simulink model "modello"  (R2022b)
settings: Solver=VariableStepAuto  StartTime=0.0  StopTime=tfinal  RelTol=1e-3
values from neighbouring files (symbols this model uses):
  A1 = [0.361538461538 0.0769230769231 0.153846153846 0.307692307692 0.272727272727 0.0818181818182 0.181818181818 0.363636363636 0.25 0.0833333333333 0.233333333333 0.333333333333 ... (16 elements, 4x4)]    [data_sim.mat]    (also in model_matrices.m = A)
  A2 = [0.4 0 0 0 0 0.5 0 0 0.4 0 0 0 ... (49 elements, 7x7)]    [data_sim.mat]    (also in model_matrices.m = A)
  A3 = [0.3 0.3 0.1 0.1 0.1 0.222222222222 0.566666666667 0 0 0.111111111111 0.5 0 ... (25 elements, 5x5)]    [data_sim.mat]    (also in model_matrices.m = A)
  A4 = [0.531578947368 0.105263157895 0.105263157895 0.105263157895 0.0526315789474 0.6 0.3 0 0 0 0.6 0 ... (25 elements, 5x5)]    [data_sim.mat]    (also in model_matrices.m = A)
  A5 = [0.566666666667 0.111111111111 0.111111111111 0.111111111111 0.6 0.3 0 0 0.5 0 0.233333333333 0.166666666667 ... (16 elements, 4x4)]    [data_sim.mat]    (also in model_matrices.m = A)
  a_0i = 0.1    [data_sim.mat]    (also in model_matrices.m)
  B1 = [1 0 0 0 0 1 0 0 0 0 1 0 ... (16 elements, 4x4)]    [data_sim.mat]    (also in model_matrices.m = eye(4))
  B2 = [1 0 0 0 0 0 0 0 1 0 0 0 ... (49 elements, 7x7)]    [data_sim.mat]    (also in model_matrices.m = eye(rn2))
  B3 = [1 0 0 0 0 0 1 0 0 0 0 0 ... (25 elements, 5x5)]    [data_sim.mat]    (also in model_matrices.m = eye(rn3))
  B4 = [1 0 0 0 0 0 1 0 0 0 0 0 ... (25 elements, 5x5)]    [data_sim.mat]    (also in model_matrices.m = eye(rn4))
  B5 = [1 0 0 0 0 1 0 0 0 0 1 0 ... (16 elements, 4x4)]    [data_sim.mat]    (also in model_matrices.m = eye(rn5))
  C1 = [1 0 0 0 0 1 0 0 0 0 1 0 ... (16 elements, 4x4)]    [data_sim.mat]    (also in model_matrices.m = eye(4))
  C2 = [1 0 0 0 0 0 0 0 1 0 0 0 ... (49 elements, 7x7)]    [data_sim.mat]    (also in model_matrices.m = eye(rn2))
  C3 = [1 0 0 0 0 0 1 0 0 0 0 0 ... (25 elements, 5x5)]    [data_sim.mat]    (also in model_matrices.m = eye(rn3))
  C4 = [1 0 0 0 0 0 1 0 0 0 0 0 ... (25 elements, 5x5)]    [data_sim.mat]    (also in model_matrices.m = eye(rn4))
  C5 = [1 0 0 0 0 1 0 0 0 0 1 0 ... (16 elements, 4x4)]    [data_sim.mat]    (also in model_matrices.m = eye(rn5))
  D1 = [0 0 0 0 0 0 0 0 0 0 0 0 ... (16 elements, 4x4)]    [data_sim.mat]    (also in model_matrices.m = zeros(4))
  D2 = [0 0 0 0 0 0 0 0 0 0 0 0 ... (49 elements, 7x7)]    [data_sim.mat]    (also in model_matrices.m = zeros(rn2))
  D3 = [0 0 0 0 0 0 0 0 0 0 0 0 ... (25 elements, 5x5)]    [data_sim.mat]    (also in model_matrices.m = zeros(rn3))
  D4 = [0 0 0 0 0 0 0 0 0 0 0 0 ... (25 elements, 5x5)]    [data_sim.mat]    (also in model_matrices.m = zeros(rn4))
  D5 = [0 0 0 0 0 0 0 0 0 0 0 0 ... (16 elements, 4x4)]    [data_sim.mat]    (also in model_matrices.m = zeros(rn5))
settings Model: Creator=Utente  LastModifiedBy=Utente

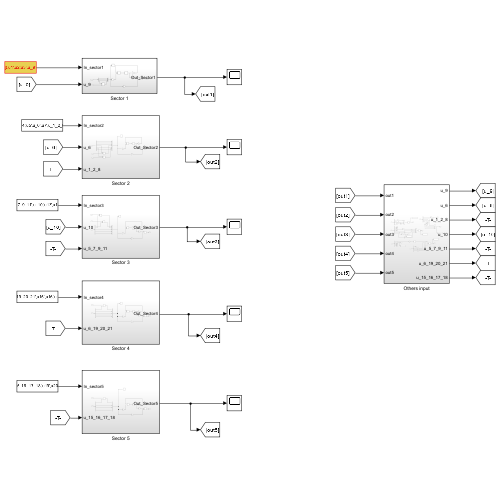
[thumbnail: Simulink's stored preview of the top-level diagram]
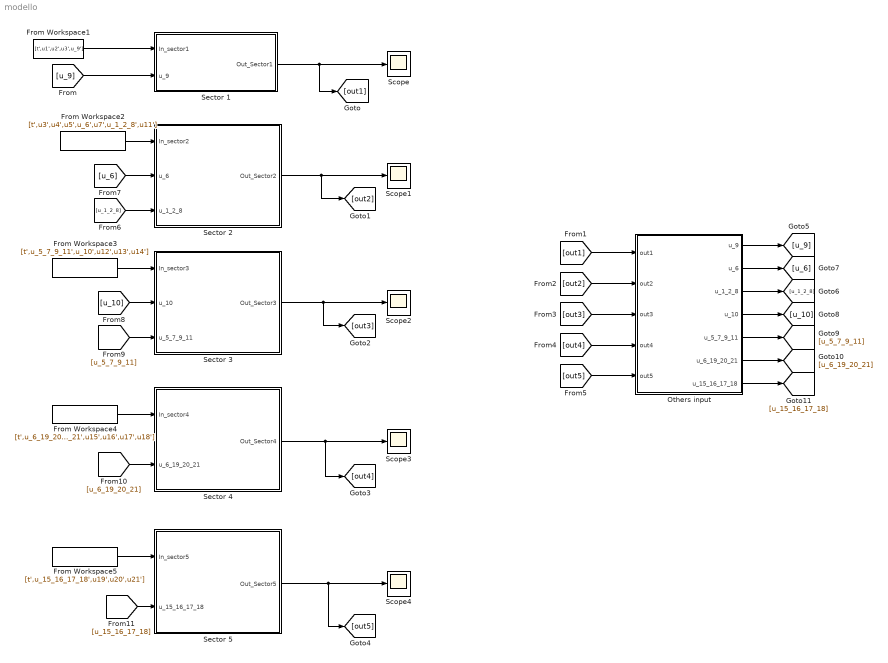
== system modello ==
  From Workspace1 : FromWorkspace  VariableName=[t',u1',u2',u3',u_9']  SampleTime=1  OutputAfterFinalValue=Holding final value
  From Workspace2 : FromWorkspace  VariableName=[t',u3',u4',u5',u_6',u7',u_1_2_8',u11']  SampleTime=1  OutputAfterFinalValue=Holding final value
  From Workspace3 : FromWorkspace  VariableName=[t',u_5_7_9_11',u_10',u12',u13',u14']  SampleTime=1  OutputAfterFinalValue=Holding final value
  From Workspace4 : FromWorkspace  VariableName=[t',u_6_19_20_21',u15',u16',u17',u18']  SampleTime=1  OutputAfterFinalValue=Holding final value
  From Workspace5 : FromWorkspace  VariableName=[t',u_15_16_17_18',u19',u20',u21']  SampleTime=1  OutputAfterFinalValue=Holding final value
  Others input : Subsystem
  Scope{,1..4} (5 alike) : Scope
  Sector 1 : Subsystem
  Sector 2 : Subsystem
  Sector 3 : Subsystem
  Sector 4 : Subsystem
  Sector 5 : Subsystem
  wires:
  Sector 1/1(Out_Sector1) -> [out1], Scope/1
  From Workspace2/1 -> Sector 2/1(In_sector2)
  Sector 2/1(Out_Sector2) -> [out2], Scope1/1
  From Workspace3/1 -> Sector 3/1(In_sector3)
  Sector 3/1(Out_Sector3) -> [out3], Scope2/1
  Sector 4/1(Out_Sector4) -> [out4], Scope3/1
  From Workspace4/1 -> Sector 4/1(In_sector4)
  From Workspace5/1 -> Sector 5/1(In_sector5)
  Sector 5/1(Out_Sector5) -> [out5], Scope4/1
  [out1] -> Others input/1(out1)
  [out2] -> Others input/2(out2)
  [out3] -> Others input/3(out3)
  [out4] -> Others input/4(out4)
  [out5] -> Others input/5(out5)
  [u_1_2_8] -> Sector 2/3(u_1_2_8)
  [u_6] -> Sector 2/2(u_6)
  [u_10] -> Sector 3/2(u_10)
  [u_5_7_9_11] -> Sector 3/3(u_5_7_9_11)
  [u_6_19_20_21] -> Sector 4/2(u_6_19_20_21)
  [u_15_16_17_18] -> Sector 5/2(u_15_16_17_18)
  Others input/1(u_9) -> [u_9]
  Others input/2(u_6) -> [u_6]
  Others input/3(u_1_2_8) -> [u_1_2_8]
  Others input/4(u_10) -> [u_10]
  Others input/5(u_5_7_9_11) -> [u_5_7_9_11]
  Others input/7(u_15_16_17_18) -> [u_15_16_17_18]
  Others input/6(u_6_19_20_21) -> [u_6_19_20_21]
  From Workspace1/1 -> Sector 1/1(In_sector1)
  [u_9] -> Sector 1/2(u_9)

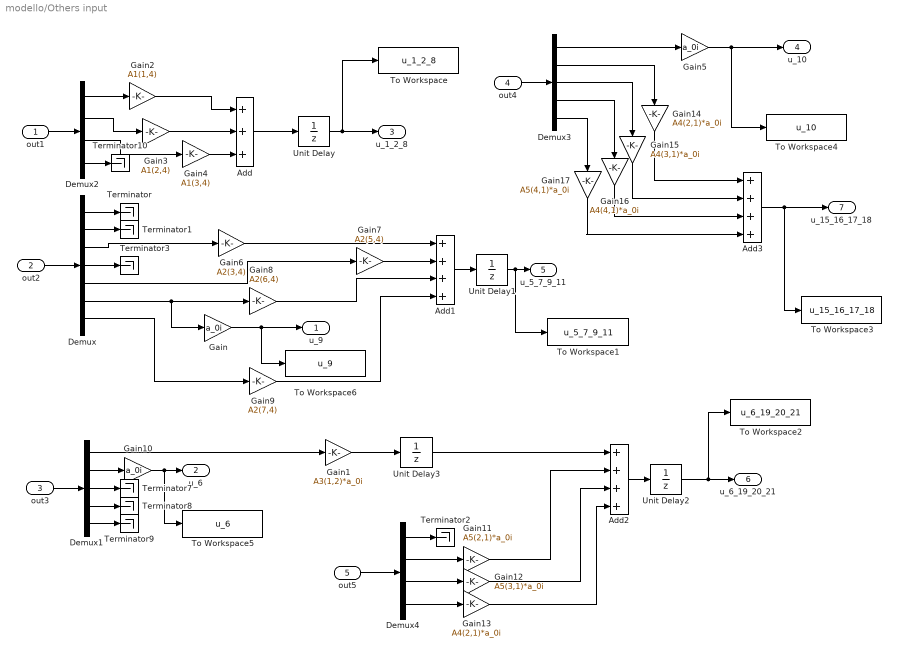
== system modello/Others input ==
  out1 : Inport
  out2 : Inport  Port=2
  out3 : Inport  Port=3
  out4 : Inport  Port=4
  out5 : Inport  Port=5
  Add : Sum  Inputs=+++
  Add1 : Sum  Inputs=++++
  Add2 : Sum  Inputs=++++
  Add3 : Sum  Inputs=++++
  Demux : Demux  Outputs=7
  Demux1 : Demux  Outputs=5
  Demux2 : Demux
  Demux3 : Demux  Outputs=5
  Demux4 : Demux
  Gain : Gain  Gain=a_0i
  Gain1 : Gain  Gain=A3(1,2)*a_0i
  Gain10 : Gain  Gain=a_0i
  Gain11 : Gain  Gain=A5(2,1)*a_0i
  Gain12 : Gain  Gain=A5(3,1)*a_0i
  Gain13 : Gain  Gain=A4(2,1)*a_0i
  Gain14 : Gain  Gain=A4(2,1)*a_0i
  Gain15 : Gain  Gain=A4(3,1)*a_0i
  Gain16 : Gain  Gain=A4(4,1)*a_0i
  Gain17 : Gain  Gain=A5(4,1)*a_0i
  Gain2 : Gain  Gain=A1(1,4)
  Gain3 : Gain  Gain=A1(2,4)
  Gain4 : Gain  Gain=A1(3,4)
  Gain5 : Gain  Gain=a_0i
  Gain6 : Gain  Gain=A2(3,4)
  Gain7 : Gain  Gain=A2(5,4)
  Gain8 : Gain  Gain=A2(6,4)
  Gain9 : Gain  Gain=A2(7,4)
  Terminator{,1..3,7..10} (8 alike) : Terminator
  To Workspace : ToWorkspace  VariableName=u_1_2_8  SampleTime=-1
  To Workspace1 : ToWorkspace  VariableName=u_5_7_9_11  SampleTime=-1
  To Workspace2 : ToWorkspace  VariableName=u_6_19_20_21  SampleTime=-1
  To Workspace3 : ToWorkspace  VariableName=u_15_16_17_18  SampleTime=-1
  To Workspace4 : ToWorkspace  VariableName=u_10  SampleTime=-1
  To Workspace5 : ToWorkspace  VariableName=u_6  SampleTime=-1
  To Workspace6 : ToWorkspace  VariableName=u_9  SampleTime=-1
  Unit Delay{,1..3} (4 alike) : UnitDelay  SampleTime=-1  HasFrameUpgradeWarning=on
  u_9 : Outport
  u_6 : Outport  Port=2
  u_1_2_8 : Outport  Port=3
  u_10 : Outport  Port=4
  u_5_7_9_11 : Outport  Port=5
  u_6_19_20_21 : Outport  Port=6
  u_15_16_17_18 : Outport  Port=7
  wires:
  Demux/6 -> Gain/1, Gain8/1
  Demux/1 -> Terminator/1
  Demux/2 -> Terminator1/1
  Demux/3 -> Gain6/1
  Demux/4 -> Terminator3/1
  Demux/5 -> Gain7/1
  Demux/7 -> Gain9/1
  Gain/1 -> To Workspace6/1, u_9/1
  out2/1 -> Demux/1
  out3/1 -> Demux1/1
  Demux1/1 -> Gain1/1
  Demux1/2 -> Gain10/1
  Demux1/3 -> Terminator7/1
  Demux1/4 -> Terminator8/1
  Demux1/5 -> Terminator9/1
  out1/1 -> Demux2/1
  Add/1 -> Unit Delay/1
  Demux2/1 -> Gain2/1
  Gain2/1 -> Add/1
  Demux2/2 -> Gain3/1
  Gain3/1 -> Add/2
  Demux2/3 -> Gain4/1
  Gain4/1 -> Add/3
  Demux2/4 -> Terminator10/1
  Demux3/5 -> Gain17/1
  Demux3/4 -> Gain16/1
  Demux3/3 -> Gain15/1
  Demux3/2 -> Gain14/1
  Demux3/1 -> Gain5/1
  Gain5/1 -> To Workspace4/1, u_10/1
  out4/1 -> Demux3/1
  Add1/1 -> Unit Delay1/1
  Gain7/1 -> Add1/2
  Gain6/1 -> Add1/1
  Gain8/1 -> Add1/3
  Gain9/1 -> Add1/4
  Add2/1 -> Unit Delay2/1
  Gain10/1 -> To Workspace5/1, u_6/1
  out5/1 -> Demux4/1
  Demux4/2 -> Gain11/1
  Gain11/1 -> Add2/2
  Demux4/3 -> Gain12/1
  Demux4/4 -> Gain13/1
  Gain12/1 -> Add2/3
  Gain13/1 -> Add2/4
  Add3/1 -> To Workspace3/1, u_15_16_17_18/1
  Gain14/1 -> Add3/1
  Gain15/1 -> Add3/2
  Gain16/1 -> Add3/3
  Gain17/1 -> Add3/4
  Unit Delay/1 -> To Workspace/1, u_1_2_8/1
  Unit Delay1/1 -> To Workspace1/1, u_5_7_9_11/1
  Unit Delay2/1 -> To Workspace2/1, u_6_19_20_21/1
  Demux4/1 -> Terminator2/1
  Gain1/1 -> Unit Delay3/1
  Unit Delay3/1 -> Add2/1

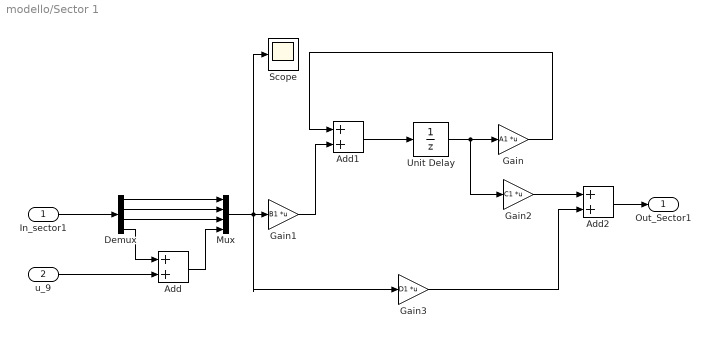
== system modello/Sector 1 ==
  In_sector1 : Inport
  u_9 : Inport  Port=2
  Add : Sum
  Add1 : Sum
  Add2 : Sum
  Demux : Demux
  Gain : Gain  Gain=A1  Multiplication=Matrix(K*u)
  Gain1 : Gain  Gain=B1  Multiplication=Matrix(K*u)
  Gain2 : Gain  Gain=C1  Multiplication=Matrix(K*u)
  Gain3 : Gain  Gain=D1  Multiplication=Matrix(K*u)
  Mux : Mux
  Scope : Scope
  Unit Delay : UnitDelay  SampleTime=-1  HasFrameUpgradeWarning=on
  Out_Sector1 : Outport
  wires:
  u_9/1 -> Add/2
  In_sector1/1 -> Demux/1
  Demux/4 -> Add/1
  Demux/1 -> Mux/1
  Demux/2 -> Mux/2
  Demux/3 -> Mux/3
  Add/1 -> Mux/4
  Unit Delay/1 -> Gain2/1, Gain/1
  Add1/1 -> Unit Delay/1
  Gain/1 -> Add1/1
  Mux/1 -> Scope/1, Gain3/1, Gain1/1
  Gain1/1 -> Add1/2
  Gain2/1 -> Add2/1
  Add2/1 -> Out_Sector1/1
  Gain3/1 -> Add2/2

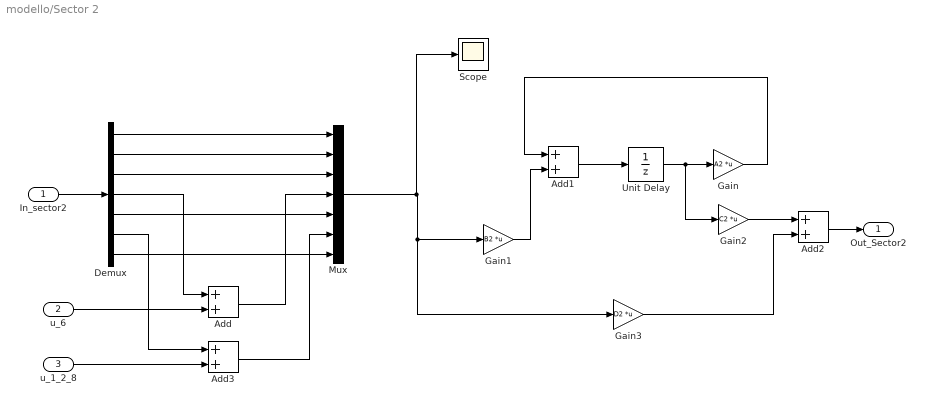
== system modello/Sector 2 ==
  In_sector2 : Inport
  u_6 : Inport  Port=2
  u_1_2_8 : Inport  Port=3
  Add{,1..3} (4 alike) : Sum
  Demux : Demux  Outputs=7
  Gain : Gain  Gain=A2  Multiplication=Matrix(K*u)
  Gain1 : Gain  Gain=B2  Multiplication=Matrix(K*u)
  Gain2 : Gain  Gain=C2  Multiplication=Matrix(K*u)
  Gain3 : Gain  Gain=D2  Multiplication=Matrix(K*u)
  Mux : Mux  Inputs=7
  Scope : Scope
  Unit Delay : UnitDelay  SampleTime=-1  HasFrameUpgradeWarning=on
  Out_Sector2 : Outport
  wires:
  Gain3/1 -> Add2/2
  Add2/1 -> Out_Sector2/1
  Gain2/1 -> Add2/1
  Mux/1 -> Scope/1, Gain1/1, Gain3/1
  Gain/1 -> Add1/1
  Add1/1 -> Unit Delay/1
  Unit Delay/1 -> Gain/1, Gain2/1
  In_sector2/1 -> Demux/1
  u_6/1 -> Add/2
  Gain1/1 -> Add1/2
  Demux/1 -> Mux/1
  Demux/2 -> Mux/2
  Demux/3 -> Mux/3
  Demux/4 -> Add/1
  Add/1 -> Mux/4
  Demux/5 -> Mux/5
  u_1_2_8/1 -> Add3/2
  Demux/7 -> Mux/7
  Demux/6 -> Add3/1
  Add3/1 -> Mux/6

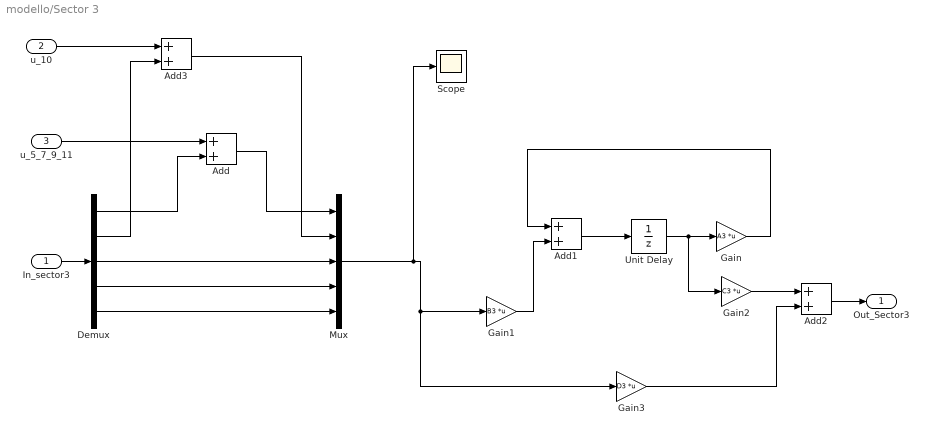
== system modello/Sector 3 ==
  In_sector3 : Inport
  u_10 : Inport  Port=2
  u_5_7_9_11 : Inport  Port=3
  Add{,1..3} (4 alike) : Sum
  Demux : Demux  Outputs=5
  Gain : Gain  Gain=A3  Multiplication=Matrix(K*u)
  Gain1 : Gain  Gain=B3  Multiplication=Matrix(K*u)
  Gain2 : Gain  Gain=C3  Multiplication=Matrix(K*u)
  Gain3 : Gain  Gain=D3  Multiplication=Matrix(K*u)
  Mux : Mux  Inputs=5
  Scope : Scope
  Unit Delay : UnitDelay  SampleTime=-1  HasFrameUpgradeWarning=on
  Out_Sector3 : Outport
  wires:
  Gain1/1 -> Add1/2
  In_sector3/1 -> Demux/1
  Unit Delay/1 -> Gain2/1, Gain/1
  Add1/1 -> Unit Delay/1
  Gain/1 -> Add1/1
  Mux/1 -> Scope/1, Gain3/1, Gain1/1
  Gain2/1 -> Add2/1
  Add2/1 -> Out_Sector3/1
  Gain3/1 -> Add2/2
  Demux/1 -> Add/2
  u_5_7_9_11/1 -> Add/1
  Add/1 -> Mux/1
  u_10/1 -> Add3/1
  Demux/2 -> Add3/2
  Add3/1 -> Mux/2
  Demux/3 -> Mux/3
  Demux/4 -> Mux/4
  Demux/5 -> Mux/5

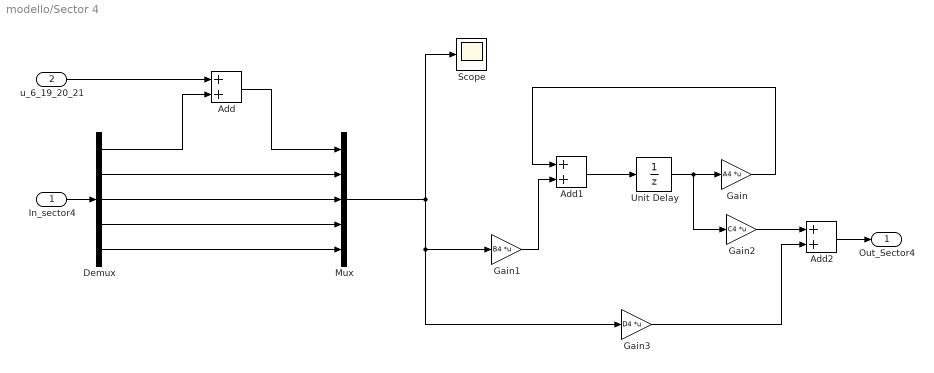
== system modello/Sector 4 ==
  In_sector4 : Inport
  u_6_19_20_21 : Inport  Port=2
  Add : Sum
  Add1 : Sum
  Add2 : Sum
  Demux : Demux  Outputs=5
  Gain : Gain  Gain=A4  Multiplication=Matrix(K*u)
  Gain1 : Gain  Gain=B4  Multiplication=Matrix(K*u)
  Gain2 : Gain  Gain=C4  Multiplication=Matrix(K*u)
  Gain3 : Gain  Gain=D4  Multiplication=Matrix(K*u)
  Mux : Mux  Inputs=5
  Scope : Scope
  Unit Delay : UnitDelay  SampleTime=-1  HasFrameUpgradeWarning=on
  Out_Sector4 : Outport
  wires:
  Gain1/1 -> Add1/2
  In_sector4/1 -> Demux/1
  Unit Delay/1 -> Gain2/1, Gain/1
  Add1/1 -> Unit Delay/1
  Gain/1 -> Add1/1
  Mux/1 -> Gain3/1, Gain1/1, Scope/1
  Gain2/1 -> Add2/1
  Add2/1 -> Out_Sector4/1
  Gain3/1 -> Add2/2
  Demux/1 -> Add/2
  u_6_19_20_21/1 -> Add/1
  Add/1 -> Mux/1
  Demux/3 -> Mux/3
  Demux/4 -> Mux/4
  Demux/5 -> Mux/5
  Demux/2 -> Mux/2

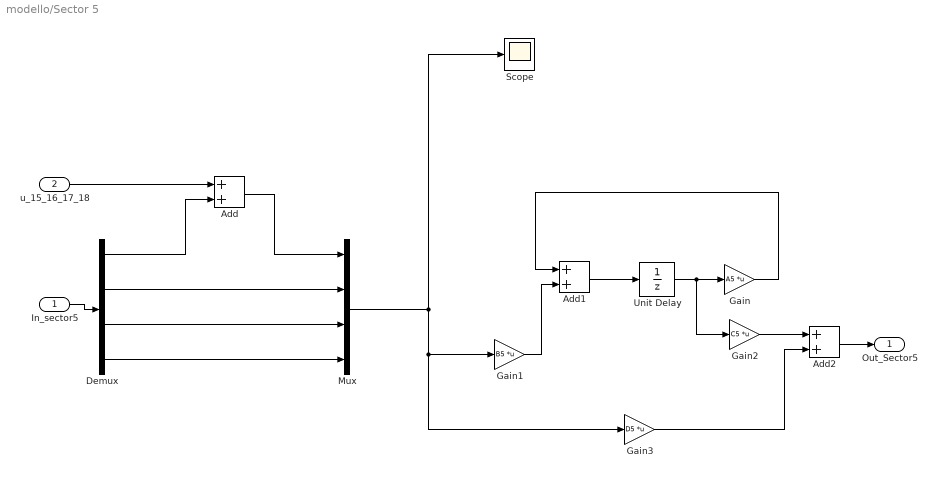
== system modello/Sector 5 ==
  In_sector5 : Inport
  u_15_16_17_18 : Inport  Port=2
  Add : Sum
  Add1 : Sum
  Add2 : Sum
  Demux : Demux
  Gain : Gain  Gain=A5  Multiplication=Matrix(K*u)
  Gain1 : Gain  Gain=B5  Multiplication=Matrix(K*u)
  Gain2 : Gain  Gain=C5  Multiplication=Matrix(K*u)
  Gain3 : Gain  Gain=D5  Multiplication=Matrix(K*u)
  Mux : Mux
  Scope : Scope
  Unit Delay : UnitDelay  SampleTime=-1  HasFrameUpgradeWarning=on
  Out_Sector5 : Outport
  wires:
  Demux/2 -> Mux/2
  Demux/4 -> Mux/4
  Demux/3 -> Mux/3
  Add/1 -> Mux/1
  u_15_16_17_18/1 -> Add/1
  Demux/1 -> Add/2
  Gain3/1 -> Add2/2
  Add2/1 -> Out_Sector5/1
  Gain2/1 -> Add2/1
  Mux/1 -> Gain1/1, Gain3/1, Scope/1
  Gain/1 -> Add1/1
  Add1/1 -> Unit Delay/1
  Unit Delay/1 -> Gain/1, Gain2/1
  In_sector5/1 -> Demux/1
  Gain1/1 -> Add1/2
